simulink model "AcasXuClosedLoop_m_1"  (R2019b)
settings: Solver=VariableStepAuto  StartTime=0.0  StopTime=30  RelTol=1e-3
libraries: neural x1560, simulink x2
(part 2 of 85)

== system AcasXuClosedLoop_m_1/networks/AcasXu_1_1/Layer 5 ==
  "a{4} " : Inport  PortDimensions=50
      mask Display: e = 0.06;c1 = [120 230 180]/255;c2 = ([120 230 180]+0)/(256+128);c3 = ([120 230 180]+128)/(256+128);patch([0 1 1 0],[0 0 1 1],c1);patch([0 1 1 1-e 1-e 0+e],[0 0 1 1-e 0+e 0+e],c2);patch([0 0 1 1-e 0+e 0+e],[0 1 1 1-e 1-e 0+e],c3);plot([0 1 1 0 0],[0 0 1 1 0]);
  Delays 1 : Subsystem
      mask Display: e = 0.06;c1 = [120 150 230]/255;c2 = ([120 150 230]+0)/383;c3 = ([120 150 230]+128)/383;patch([0 1 1 0],[0 0 1 1],c1);patch([0 1 1 1-e 1-e 0+e],[0 0 1 1-e 0+e 0+e],c2);patch([0 0 1 1-e 0+e 0+e],[0 1 1 1-e 1-e 0+e],c3);plot([0 1 1 0 0],[0 0 1 1 0]);disp('0');
  "LW{5,4}" : Subsystem
      mask Display: e = 0.06;c1 = [120 150 230]/255;c2 = ([120 150 230]+0)/383;c3 = ([120 150 230]+128)/383;patch([0 1 1 0],[0 0 1 1],c1);patch([0 1 1 1-e 1-e 0+e],[0 0 1 1-e 0+e 0+e],c2);patch([0 0 1 1-e 0+e 0+e],[0 1 1 1-e 1-e 0+e],c3);plot([0 1 1 0 0],[0 0 1 1 0]);disp('W');
  "b{5}" : Constant  Value=[0.343884000000000022989610215518041513860225677490234375;-0.148704000000000002845723656719201244413852691650390625;-0.182344000000000006078693104427657090127468109130859375;2.092820000000000124629195852321572601795196533203125;0.057392100000000001447375552743324078619480133056640625;1.0727800000000000668620714350254274904727935791015625;-3.537500000000000088817841970012523233890533447265625;0.2902460000000000039932501749717630445957183837890625;1.7852799999999999780442294650129042565822601318359375;0.5703920000000000101181285572238266468048095703125;0.102578000000000002511768570911954157054424285888671875;-0.8676939999999999653113036401919089257717132568359375;-1.8884399999999998964739233997534029185771942138671875;-1.11488999999999993661958797019906342029571533203125;-0.445674999999999987831955650108284316956996917724609375;0.694015999999999966263430906110443174839019775390625;1.2776199999999999779021209178608842194080352783203125;-1.2911200000000000454036808150704018771648406982421875;-1.34224999999999994315658113919198513031005859375;-0.15967100000000000736832816983223892748355865478515625;0.64522299999999999098321268320432864129543304443359375;0.988628999999999980019538270425982773303985595703125;0.5161510000000000264464006249909289181232452392578125;-2.3827400000000000801492205937393009662628173828125;0.67675600000000002420819100734661333262920379638671875;0.76186699999999996091304410583688877522945404052734375;0.056760600000000001330580090552757610566914081573486328125;-0.2224609999999999920827775667930836789309978485107421875;1.869569999999999954098939269897527992725372314453125;1.052049999999999929656269159750081598758697509765625;-0.1076290000000000024460433678541448898613452911376953125;0.0906623000000000012210676914037321694195270538330078125;2.556319999999999925677229839493520557880401611328125;0.87517400000000000748201500755385495722293853759765625;0.08279160000000000685371759345798636786639690399169921875;-1.1624499999999999833022457096376456320285797119140625;1.1968300000000000604671868131845258176326751708984375;0.11945899999999999574473719121670001186430454254150390625;0.052382600000000001383426706524915061891078948974609375;-0.25143999999999999683808482586755417287349700927734375;0.9712009999999999809716655363445170223712921142578125;0.41452299999999997481836544466204941272735595703125;0.55931600000000003536371195878018625080585479736328125;0.71126500000000003609557097661308944225311279296875;-3.244779999999999997584154698415659368038177490234375;0.57999999999999996003197111349436454474925994873046875;0.165872999999999992670751680634566582739353179931640625;-1.2932699999999999196376165855326689779758453369140625;-0.331040999999999974168218841441557742655277252197265625;-0.65416499999999999648281345798750407993793487548828125]
      mask Display: e = 0.06;c1 = [120 150 230]/255;c2 = ([120 150 230]+0)/383;c3 = ([120 150 230]+128)/383;patch([0 1 1 0],[0 0 1 1],c1);patch([0 1 1 1-e 1-e 0+e],[0 0 1 1-e 0+e 0+e],c2);patch([0 0 1 1-e 0+e 0+e],[0 1 1 1-e 1-e 0+e],c3);plot([0 1 1 0 0],[0 0 1 1 0]);disp('b');
  netsum : Sum  Inputs=2  SaturateOnIntegerOverflow=on  InputSameDT=on  OutDataTypeStr=Inherit: Same as first input
      mask Display: e = 0.06;c1 = [120 150 230]/255;c2 = ([120 150 230]+0)/383;c3 = ([120 150 230]+128)/383;patch([0 1 1 0],[0 0 1 1],c1);patch([0 1 1 1-e 1-e 0+e],[0 0 1 1-e 0+e 0+e],c2);patch([0 0 1 1-e 0+e 0+e],[0 1 1 1-e 1-e 0+e],c3);plot([0 1 1 0 0],[0 0 1 1 0]);disp('+');
  tansig : neural/Transfer Functions/tansig
      settings: SourceProductName=Deep Learning Toolbox
  "a{5}" : Outport  InitialOutput=[0;0;0;0;0;0;0;0;0;0;0;0;0;0;0;0;0;0;0;0;0;0;0;0;0;0;0;0;0;0;0;0;0;0;0;0;0;0;0;0;0;0;0;0;0;0;0;0;0;0]
      mask Display: e = 0.06;c1 = [120 230 180]/255;c2 = ([120 230 180]+0)/(256+128);c3 = ([120 230 180]+128)/(256+128);patch([0 1 1 0],[0 0 1 1],c1);patch([0 1 1 1-e 1-e 0+e],[0 0 1 1-e 0+e 0+e],c2);patch([0 0 1 1-e 0+e 0+e],[0 1 1 1-e 1-e 0+e],c3);plot([0 1 1 0 0],[0 0 1 1 0]);
  wires:
  tansig/1 -> "a{5}"/1
  netsum/1 -> tansig/1
  "b{5}"/1 -> netsum/2
  "LW{5,4}"/1("lz{5,4}") -> netsum/1
  Delays 1/1("pd{5,4}") -> "LW{5,4}"/1("ad{5,4}")
  "a{4} "/1 -> Delays 1/1("p{5}")

== system AcasXuClosedLoop_m_1/networks/AcasXu_1_1/Layer 6 ==
  "a{5} " : Inport  PortDimensions=50
      mask Display: e = 0.06;c1 = [120 230 180]/255;c2 = ([120 230 180]+0)/(256+128);c3 = ([120 230 180]+128)/(256+128);patch([0 1 1 0],[0 0 1 1],c1);patch([0 1 1 1-e 1-e 0+e],[0 0 1 1-e 0+e 0+e],c2);patch([0 0 1 1-e 0+e 0+e],[0 1 1 1-e 1-e 0+e],c3);plot([0 1 1 0 0],[0 0 1 1 0]);
  Delays 1 : Subsystem
      mask Display: e = 0.06;c1 = [120 150 230]/255;c2 = ([120 150 230]+0)/383;c3 = ([120 150 230]+128)/383;patch([0 1 1 0],[0 0 1 1],c1);patch([0 1 1 1-e 1-e 0+e],[0 0 1 1-e 0+e 0+e],c2);patch([0 0 1 1-e 0+e 0+e],[0 1 1 1-e 1-e 0+e],c3);plot([0 1 1 0 0],[0 0 1 1 0]);disp('0');
  "LW{6,5}" : Subsystem
      mask Display: e = 0.06;c1 = [120 150 230]/255;c2 = ([120 150 230]+0)/383;c3 = ([120 150 230]+128)/383;patch([0 1 1 0],[0 0 1 1],c1);patch([0 1 1 1-e 1-e 0+e],[0 0 1 1-e 0+e 0+e],c2);patch([0 0 1 1-e 0+e 0+e],[0 1 1 1-e 1-e 0+e],c3);plot([0 1 1 0 0],[0 0 1 1 0]);disp('W');
  "b{6}" : Constant  Value=[-0.4300610000000000265885091721429489552974700927734375;-0.0245742000000000009041212223337424802593886852264404296875;-1.857369999999999965467623042059130966663360595703125;-0.0138151999999999997026378650843980722129344940185546875;0.419246999999999980790477138725691474974155426025390625;-0.2135869999999999990780708003512700088322162628173828125;0.160069999999999990070165267752599902451038360595703125;0.741837999999999997413624441833235323429107666015625;0.0084694499999999998951505375544002163223922252655029296875;-0.72603399999999995717558931573876179754734039306640625;-4.7420600000000003859668140648864209651947021484375;0.069490200000000001967492835319717414677143096923828125;-0.332739999999999980229148377475212328135967254638671875;0.4584289999999999754010104879853315651416778564453125;-1.0340100000000000957101065068854950368404388427734375;-0.436593999999999982097875772524275816977024078369140625;0.08706809999999999549746831917218514718115329742431640625;-1.1747900000000000009237055564881302416324615478515625;0.29503800000000002246025587737676687538623809814453125;0.648179999999999978399500832892954349517822265625;0.59697699999999997988453515063156373798847198486328125;-2.17555999999999993832489053602330386638641357421875;-1.1105899999999999661071115042432211339473724365234375;-0.429719000000000017625012560529285110533237457275390625;0.241839999999999999413802242997917346656322479248046875;0.161131999999999997452704292300040833652019500732421875;0.10325099999999999555999607991907396353781223297119140625;0.1906210000000000126529897670479840599000453948974609375;-2.56280999999999981042719809920527040958404541015625;0.428493999999999986005860819204826839268207550048828125;0.1659190000000000109192654917933396063745021820068359375;-0.041315499999999998059774242165076429955661296844482421875;-3.21201999999999987522869560052640736103057861328125;0.0165723000000000016129764190964124281890690326690673828125;-1.449510000000000076170181273482739925384521484375;-0.212716999999999989423571378210908733308315277099609375;0.096362000000000003208100451956852339208126068115234375;-0.1836109999999999964348518233236973173916339874267578125;-0.55453399999999997138644403094076551496982574462890625;0.33988600000000002143707433788222260773181915283203125;0.366640000000000021440627051561023108661174774169921875;1.1872499999999999165112285481882281601428985595703125;-7.00659999999999971720399116748012602329254150390625;0.8648160000000000291464630208793096244335174560546875;-4.08664999999999967172925607883371412754058837890625;0.1906569999999999931450389567544334568083286285400390625;0.438983999999999985330845220232731662690639495849609375;-0.66478899999999996328625684327562339603900909423828125;-0.1143470000000000041939784978239913471043109893798828125;0.12170599999999999474287193379495874978601932525634765625]
      mask Display: e = 0.06;c1 = [120 150 230]/255;c2 = ([120 150 230]+0)/383;c3 = ([120 150 230]+128)/383;patch([0 1 1 0],[0 0 1 1],c1);patch([0 1 1 1-e 1-e 0+e],[0 0 1 1-e 0+e 0+e],c2);patch([0 0 1 1-e 0+e 0+e],[0 1 1 1-e 1-e 0+e],c3);plot([0 1 1 0 0],[0 0 1 1 0]);disp('b');
  netsum : Sum  Inputs=2  SaturateOnIntegerOverflow=on  InputSameDT=on  OutDataTypeStr=Inherit: Same as first input
      mask Display: e = 0.06;c1 = [120 150 230]/255;c2 = ([120 150 230]+0)/383;c3 = ([120 150 230]+128)/383;patch([0 1 1 0],[0 0 1 1],c1);patch([0 1 1 1-e 1-e 0+e],[0 0 1 1-e 0+e 0+e],c2);patch([0 0 1 1-e 0+e 0+e],[0 1 1 1-e 1-e 0+e],c3);plot([0 1 1 0 0],[0 0 1 1 0]);disp('+');
  tansig : neural/Transfer Functions/tansig
      settings: SourceProductName=Deep Learning Toolbox
  "a{6}" : Outport  InitialOutput=[0;0;0;0;0;0;0;0;0;0;0;0;0;0;0;0;0;0;0;0;0;0;0;0;0;0;0;0;0;0;0;0;0;0;0;0;0;0;0;0;0;0;0;0;0;0;0;0;0;0]
      mask Display: e = 0.06;c1 = [120 230 180]/255;c2 = ([120 230 180]+0)/(256+128);c3 = ([120 230 180]+128)/(256+128);patch([0 1 1 0],[0 0 1 1],c1);patch([0 1 1 1-e 1-e 0+e],[0 0 1 1-e 0+e 0+e],c2);patch([0 0 1 1-e 0+e 0+e],[0 1 1 1-e 1-e 0+e],c3);plot([0 1 1 0 0],[0 0 1 1 0]);
  wires:
  tansig/1 -> "a{6}"/1
  netsum/1 -> tansig/1
  "b{6}"/1 -> netsum/2
  "LW{6,5}"/1("lz{6,5}") -> netsum/1
  Delays 1/1("pd{6,5}") -> "LW{6,5}"/1("ad{6,5}")
  "a{5} "/1 -> Delays 1/1("p{6}")

== system AcasXuClosedLoop_m_1/networks/AcasXu_1_1/Layer 7 ==
  "a{6} " : Inport  PortDimensions=50
      mask Display: e = 0.06;c1 = [120 230 180]/255;c2 = ([120 230 180]+0)/(256+128);c3 = ([120 230 180]+128)/(256+128);patch([0 1 1 0],[0 0 1 1],c1);patch([0 1 1 1-e 1-e 0+e],[0 0 1 1-e 0+e 0+e],c2);patch([0 0 1 1-e 0+e 0+e],[0 1 1 1-e 1-e 0+e],c3);plot([0 1 1 0 0],[0 0 1 1 0]);
  Delays 1 : Subsystem
      mask Display: e = 0.06;c1 = [120 150 230]/255;c2 = ([120 150 230]+0)/383;c3 = ([120 150 230]+128)/383;patch([0 1 1 0],[0 0 1 1],c1);patch([0 1 1 1-e 1-e 0+e],[0 0 1 1-e 0+e 0+e],c2);patch([0 0 1 1-e 0+e 0+e],[0 1 1 1-e 1-e 0+e],c3);plot([0 1 1 0 0],[0 0 1 1 0]);disp('0');
  "LW{7,6}" : Subsystem
      mask Display: e = 0.06;c1 = [120 150 230]/255;c2 = ([120 150 230]+0)/383;c3 = ([120 150 230]+128)/383;patch([0 1 1 0],[0 0 1 1],c1);patch([0 1 1 1-e 1-e 0+e],[0 0 1 1-e 0+e 0+e],c2);patch([0 0 1 1-e 0+e 0+e],[0 1 1 1-e 1-e 0+e],c3);plot([0 1 1 0 0],[0 0 1 1 0]);disp('W');
  "b{7}" : Constant  Value=[-0.01028150000000000070798922280346232582814991474151611328125;-0.01586680000000000034798830483850906603038311004638671875;-0.01548229999999999918769422180275796563364565372467041015625;-0.01533600000000000067312821983023241045884788036346435546875;-0.0148281000000000003080646848729884368367493152618408203125]
      mask Display: e = 0.06;c1 = [120 150 230]/255;c2 = ([120 150 230]+0)/383;c3 = ([120 150 230]+128)/383;patch([0 1 1 0],[0 0 1 1],c1);patch([0 1 1 1-e 1-e 0+e],[0 0 1 1-e 0+e 0+e],c2);patch([0 0 1 1-e 0+e 0+e],[0 1 1 1-e 1-e 0+e],c3);plot([0 1 1 0 0],[0 0 1 1 0]);disp('b');
  netsum : Sum  Inputs=2  SaturateOnIntegerOverflow=on  InputSameDT=on  OutDataTypeStr=Inherit: Same as first input
      mask Display: e = 0.06;c1 = [120 150 230]/255;c2 = ([120 150 230]+0)/383;c3 = ([120 150 230]+128)/383;patch([0 1 1 0],[0 0 1 1],c1);patch([0 1 1 1-e 1-e 0+e],[0 0 1 1-e 0+e 0+e],c2);patch([0 0 1 1-e 0+e 0+e],[0 1 1 1-e 1-e 0+e],c3);plot([0 1 1 0 0],[0 0 1 1 0]);disp('+');
  purelin : neural/Transfer Functions/purelin
      settings: SourceProductName=Deep Learning Toolbox
  "a{7}" : Outport  InitialOutput=[0;0;0;0;0]
      mask Display: e = 0.06;c1 = [120 230 180]/255;c2 = ([120 230 180]+0)/(256+128);c3 = ([120 230 180]+128)/(256+128);patch([0 1 1 0],[0 0 1 1],c1);patch([0 1 1 1-e 1-e 0+e],[0 0 1 1-e 0+e 0+e],c2);patch([0 0 1 1-e 0+e 0+e],[0 1 1 1-e 1-e 0+e],c3);plot([0 1 1 0 0],[0 0 1 1 0]);
  wires:
  purelin/1 -> "a{7}"/1
  netsum/1 -> purelin/1
  "b{7}"/1 -> netsum/2
  "LW{7,6}"/1("lz{7,6}") -> netsum/1
  Delays 1/1("pd{7,6}") -> "LW{7,6}"/1("ad{7,6}")
  "a{6} "/1 -> Delays 1/1("p{7}")

== system AcasXuClosedLoop_m_1/networks/AcasXu_1_1/Process Input 1 ==
  x : Inport  PortDimensions=5
      mask Display: e = 0.06;c1 = [120 230 180]/255;c2 = ([120 230 180]+0)/(256+128);c3 = ([120 230 180]+128)/(256+128);patch([0 1 1 0],[0 0 1 1],c1);patch([0 1 1 1-e 1-e 0+e],[0 0 1 1-e 0+e 0+e],c2);patch([0 0 1 1-e 0+e 0+e],[0 1 1 1-e 1-e 0+e],c3);plot([0 1 1 0 0],[0 0 1 1 0]);
  p : Outport  PortDimensions=5
      mask Display: e = 0.06;c1 = [120 230 180]/255;c2 = ([120 230 180]+0)/(256+128);c3 = ([120 230 180]+128)/(256+128);patch([0 1 1 0],[0 0 1 1],c1);patch([0 1 1 1-e 1-e 0+e],[0 0 1 1-e 0+e 0+e],c2);patch([0 0 1 1-e 0+e 0+e],[0 1 1 1-e 1-e 0+e],c3);plot([0 1 1 0 0],[0 0 1 1 0]);
  wires:
  x/1 -> p/1

== system AcasXuClosedLoop_m_1/networks/AcasXu_1_1/Process Output 1 ==
  a : Inport  PortDimensions=5
      mask Display: e = 0.06;c1 = [120 230 180]/255;c2 = ([120 230 180]+0)/(256+128);c3 = ([120 230 180]+128)/(256+128);patch([0 1 1 0],[0 0 1 1],c1);patch([0 1 1 1-e 1-e 0+e],[0 0 1 1-e 0+e 0+e],c2);patch([0 0 1 1-e 0+e 0+e],[0 1 1 1-e 1-e 0+e],c3);plot([0 1 1 0 0],[0 0 1 1 0]);
  y : Outport  PortDimensions=5
      mask Display: e = 0.06;c1 = [120 230 180]/255;c2 = ([120 230 180]+0)/(256+128);c3 = ([120 230 180]+128)/(256+128);patch([0 1 1 0],[0 0 1 1],c1);patch([0 1 1 1-e 1-e 0+e],[0 0 1 1-e 0+e 0+e],c2);patch([0 0 1 1-e 0+e 0+e],[0 1 1 1-e 1-e 0+e],c3);plot([0 1 1 0 0],[0 0 1 1 0]);
  wires:
  a/1 -> y/1

== system AcasXuClosedLoop_m_1/networks/AcasXu_2_1/Layer 1 ==
  "p{1}" : Inport  PortDimensions=5
      mask Display: e = 0.06;c1 = [120 230 180]/255;c2 = ([120 230 180]+0)/(256+128);c3 = ([120 230 180]+128)/(256+128);patch([0 1 1 0],[0 0 1 1],c1);patch([0 1 1 1-e 1-e 0+e],[0 0 1 1-e 0+e 0+e],c2);patch([0 0 1 1-e 0+e 0+e],[0 1 1 1-e 1-e 0+e],c3);plot([0 1 1 0 0],[0 0 1 1 0]);
  Delays 1 : Subsystem
      mask Display: e = 0.06;c1 = [120 150 230]/255;c2 = ([120 150 230]+0)/383;c3 = ([120 150 230]+128)/383;patch([0 1 1 0],[0 0 1 1],c1);patch([0 1 1 1-e 1-e 0+e],[0 0 1 1-e 0+e 0+e],c2);patch([0 0 1 1-e 0+e 0+e],[0 1 1 1-e 1-e 0+e],c3);plot([0 1 1 0 0],[0 0 1 1 0]);disp('0');
  "IW{1,1}" : Subsystem
      mask Display: e = 0.06;c1 = [120 150 230]/255;c2 = ([120 150 230]+0)/383;c3 = ([120 150 230]+128)/383;patch([0 1 1 0],[0 0 1 1],c1);patch([0 1 1 1-e 1-e 0+e],[0 0 1 1-e 0+e 0+e],c2);patch([0 0 1 1-e 0+e 0+e],[0 1 1 1-e 1-e 0+e],c3);plot([0 1 1 0 0],[0 0 1 1 0]);disp('W');
  "b{1}" : Constant  Value=[0.1625659999999999882902557146735489368438720703125;-0.5818280000000000118376419777632690966129302978515625;-0.8015470000000000094786400950397364795207977294921875;-0.030902499999999999413802242997917346656322479248046875;-0.80615000000000003321787289678468368947505950927734375;-0.044919300000000002281996813735531759448349475860595703125;0.39823100000000000164845914696343243122100830078125;-0.01291710000000000080344619846073328517377376556396484375;-0.15108800000000000007815970093361102044582366943359375;-0.08336590000000000666435795437791966833174228668212890625;0.01728899999999999881339363128063268959522247314453125;0.276963999999999987977616910939104855060577392578125;-0.1317879999999999884874313238469767384231090545654296875;0.1621620000000000005879741138414829038083553314208984375;0.09520820000000000671303013177748653106391429901123046875;-0.50132100000000001660538373471354134380817413330078125;-0.31888600000000000278532752417959272861480712890625;-0.0747223999999999943799622315054875798523426055908203125;-0.467965000000000019841905896100797690451145172119140625;-0.1974539999999999906332703858424792997539043426513671875;-0.12473700000000000065458749531899229623377323150634765625;-0.16273199999999998777155951756867580115795135498046875;-0.0641459000000000056918025848062825389206409454345703125;0.2065120000000000011208811656615580432116985321044921875;-0.2566800000000000192557081390987150371074676513671875;0.1934780000000000110826903210181626491248607635498046875;-0.9121580000000000243431941271410323679447174072265625;0.00345349999999999997257749129175863345153629779815673828125;-0.29590199999999999835864628039416857063770294189453125;-0.7066689999999999916013848633156158030033111572265625;0.051531500000000000916156039920679177157580852508544921875;-0.100573999999999996735056129182339645922183990478515625;-0.11314000000000000445421477479612804017961025238037109375;-0.68570600000000003770850298678851686418056488037109375;-0.75538199999999999789679350215010344982147216796875;0.61229900000000003768008127735811285674571990966796875;0.0901586000000000054033222340876818634569644927978515625;-0.477876000000000022982504788160440512001514434814453125;-0.06931059999999999998721023075631819665431976318359375;-0.63012400000000001742961330819525755941867828369140625;-0.49970700000000001228528390129213221371173858642578125;0.155584000000000000074606987254810519516468048095703125;-0.36052899999999998836841541560715995728969573974609375;0.0822959000000000051588955329862073995172977447509765625;-0.046897899999999999309796550051032681949436664581298828125;0.053298900000000003218669775151283829472959041595458984375;0.44651099999999999123900806807796470820903778076171875;-0.460731999999999974892972431916859932243824005126953125;0.1620850000000000068478556158879655413329601287841796875;-0.6189270000000000049311665861750952899456024169921875]
      mask Display: e = 0.06;c1 = [120 150 230]/255;c2 = ([120 150 230]+0)/383;c3 = ([120 150 230]+128)/383;patch([0 1 1 0],[0 0 1 1],c1);patch([0 1 1 1-e 1-e 0+e],[0 0 1 1-e 0+e 0+e],c2);patch([0 0 1 1-e 0+e 0+e],[0 1 1 1-e 1-e 0+e],c3);plot([0 1 1 0 0],[0 0 1 1 0]);disp('b');
  netsum : Sum  Inputs=2  SaturateOnIntegerOverflow=on  InputSameDT=on  OutDataTypeStr=Inherit: Same as first input
      mask Display: e = 0.06;c1 = [120 150 230]/255;c2 = ([120 150 230]+0)/383;c3 = ([120 150 230]+128)/383;patch([0 1 1 0],[0 0 1 1],c1);patch([0 1 1 1-e 1-e 0+e],[0 0 1 1-e 0+e 0+e],c2);patch([0 0 1 1-e 0+e 0+e],[0 1 1 1-e 1-e 0+e],c3);plot([0 1 1 0 0],[0 0 1 1 0]);disp('+');
  tansig : neural/Transfer Functions/tansig
      settings: SourceProductName=Deep Learning Toolbox
  "a{1}" : Outport  InitialOutput=[0;0;0;0;0;0;0;0;0;0;0;0;0;0;0;0;0;0;0;0;0;0;0;0;0;0;0;0;0;0;0;0;0;0;0;0;0;0;0;0;0;0;0;0;0;0;0;0;0;0]
      mask Display: e = 0.06;c1 = [120 230 180]/255;c2 = ([120 230 180]+0)/(256+128);c3 = ([120 230 180]+128)/(256+128);patch([0 1 1 0],[0 0 1 1],c1);patch([0 1 1 1-e 1-e 0+e],[0 0 1 1-e 0+e 0+e],c2);patch([0 0 1 1-e 0+e 0+e],[0 1 1 1-e 1-e 0+e],c3);plot([0 1 1 0 0],[0 0 1 1 0]);
  wires:
  tansig/1 -> "a{1}"/1
  netsum/1 -> tansig/1
  "b{1}"/1 -> netsum/2
  "IW{1,1}"/1("iz{1,1}") -> netsum/1
  Delays 1/1("pd{1,1}") -> "IW{1,1}"/1("pd{1,1}")
  "p{1}"/1 -> Delays 1/1("p{1}")

== system AcasXuClosedLoop_m_1/networks/AcasXu_2_1/Layer 2 ==
  "a{1} " : Inport  PortDimensions=50
      mask Display: e = 0.06;c1 = [120 230 180]/255;c2 = ([120 230 180]+0)/(256+128);c3 = ([120 230 180]+128)/(256+128);patch([0 1 1 0],[0 0 1 1],c1);patch([0 1 1 1-e 1-e 0+e],[0 0 1 1-e 0+e 0+e],c2);patch([0 0 1 1-e 0+e 0+e],[0 1 1 1-e 1-e 0+e],c3);plot([0 1 1 0 0],[0 0 1 1 0]);
  Delays 1 : Subsystem
      mask Display: e = 0.06;c1 = [120 150 230]/255;c2 = ([120 150 230]+0)/383;c3 = ([120 150 230]+128)/383;patch([0 1 1 0],[0 0 1 1],c1);patch([0 1 1 1-e 1-e 0+e],[0 0 1 1-e 0+e 0+e],c2);patch([0 0 1 1-e 0+e 0+e],[0 1 1 1-e 1-e 0+e],c3);plot([0 1 1 0 0],[0 0 1 1 0]);disp('0');
  "LW{2,1}" : Subsystem
      mask Display: e = 0.06;c1 = [120 150 230]/255;c2 = ([120 150 230]+0)/383;c3 = ([120 150 230]+128)/383;patch([0 1 1 0],[0 0 1 1],c1);patch([0 1 1 1-e 1-e 0+e],[0 0 1 1-e 0+e 0+e],c2);patch([0 0 1 1-e 0+e 0+e],[0 1 1 1-e 1-e 0+e],c3);plot([0 1 1 0 0],[0 0 1 1 0]);disp('W');
  "b{2}" : Constant  Value=[0.552667000000000019355184122105129063129425048828125;-0.6503900000000000236610731008113361895084381103515625;0.7978330000000000143955958264996297657489776611328125;-0.36217500000000002469136006766348145902156829833984375;0.61262600000000000388666876460774801671504974365234375;0.752850000000000019184653865522705018520355224609375;-0.1222810000000000008046896482483134604990482330322265625;-0.004129449999999999787458904165760031901299953460693359375;-0.141452999999999995406341213310952298343181610107421875;-0.656487999999999960465402182308025658130645751953125;0.2476059999999999927666749499621801078319549560546875;-0.0221704999999999992355004252431172062642872333526611328125;0.7398270000000000123918653116561472415924072265625;-0.226283000000000011908696251339279115200042724609375;0.94933999999999996166621940574259497225284576416015625;-0.005919210000000000269915201300818807794712483882904052734375;-0.60101899999999996992983142263256013393402099609375;-0.2269480000000000108340003635021275840699672698974609375;1.03943999999999991956656231195665895938873291015625;-0.056692499999999999837907438404727145098149776458740234375;-0.91461599999999998455990635193302296102046966552734375;0.1633320000000000049578119387660990469157695770263671875;0.304910000000000014352963262354023754596710205078125;-0.70832200000000000716937620381941087543964385986328125;1.278799999999999936761696517351083457469940185546875;1.052869999999999972573050399660132825374603271484375;-0.225430999999999992500221424052142538130283355712890625;-0.2357329999999999980975218250023317523300647735595703125;0.14560899999999998843946968918316997587680816650390625;0.79074999999999995292654375589336268603801727294921875;-0.006529100000000000354749563058476269361563026905059814453125;0.60662000000000004806821607417077757418155670166015625;-0.67515800000000003588951358324266038835048675537109375;0.68973700000000004450839696801267564296722412109375;-0.039575800000000001255262560562186990864574909210205078125;0.026829300000000000370192765331012196838855743408203125;-0.4289330000000000087112539404188282787799835205078125;-0.0243698000000000004894307181757540092803537845611572265625;-1.28910999999999997811528373858891427516937255859375;-0.2416580000000000116866516464142478071153163909912109375;-0.376342000000000009851675031313789077103137969970703125;-0.124746999999999996777688693327945657074451446533203125;-0.287582999999999977536191408944432623684406280517578125;-0.413968999999999975880626834623399190604686737060546875;0.09448620000000000629380991767902742139995098114013671875;0.162760999999999989018562018827651627361774444580078125;-0.340011000000000007670308832530281506478786468505859375;-0.40002999999999999669597627871553413569927215576171875;0.4314810000000000034248159863636828958988189697265625;-1.514089999999999935909045234438963234424591064453125]
      mask Display: e = 0.06;c1 = [120 150 230]/255;c2 = ([120 150 230]+0)/383;c3 = ([120 150 230]+128)/383;patch([0 1 1 0],[0 0 1 1],c1);patch([0 1 1 1-e 1-e 0+e],[0 0 1 1-e 0+e 0+e],c2);patch([0 0 1 1-e 0+e 0+e],[0 1 1 1-e 1-e 0+e],c3);plot([0 1 1 0 0],[0 0 1 1 0]);disp('b');
  netsum : Sum  Inputs=2  SaturateOnIntegerOverflow=on  InputSameDT=on  OutDataTypeStr=Inherit: Same as first input
      mask Display: e = 0.06;c1 = [120 150 230]/255;c2 = ([120 150 230]+0)/383;c3 = ([120 150 230]+128)/383;patch([0 1 1 0],[0 0 1 1],c1);patch([0 1 1 1-e 1-e 0+e],[0 0 1 1-e 0+e 0+e],c2);patch([0 0 1 1-e 0+e 0+e],[0 1 1 1-e 1-e 0+e],c3);plot([0 1 1 0 0],[0 0 1 1 0]);disp('+');
  tansig : neural/Transfer Functions/tansig
      settings: SourceProductName=Deep Learning Toolbox
  "a{2}" : Outport  InitialOutput=[0;0;0;0;0;0;0;0;0;0;0;0;0;0;0;0;0;0;0;0;0;0;0;0;0;0;0;0;0;0;0;0;0;0;0;0;0;0;0;0;0;0;0;0;0;0;0;0;0;0]
      mask Display: e = 0.06;c1 = [120 230 180]/255;c2 = ([120 230 180]+0)/(256+128);c3 = ([120 230 180]+128)/(256+128);patch([0 1 1 0],[0 0 1 1],c1);patch([0 1 1 1-e 1-e 0+e],[0 0 1 1-e 0+e 0+e],c2);patch([0 0 1 1-e 0+e 0+e],[0 1 1 1-e 1-e 0+e],c3);plot([0 1 1 0 0],[0 0 1 1 0]);
  wires:
  tansig/1 -> "a{2}"/1
  netsum/1 -> tansig/1
  "b{2}"/1 -> netsum/2
  "LW{2,1}"/1("lz{2,1}") -> netsum/1
  Delays 1/1("pd{2,1}") -> "LW{2,1}"/1("ad{2,1}")
  "a{1} "/1 -> Delays 1/1("p{2}")

== system AcasXuClosedLoop_m_1/networks/AcasXu_2_1/Layer 3 ==
  "a{2} " : Inport  PortDimensions=50
      mask Display: e = 0.06;c1 = [120 230 180]/255;c2 = ([120 230 180]+0)/(256+128);c3 = ([120 230 180]+128)/(256+128);patch([0 1 1 0],[0 0 1 1],c1);patch([0 1 1 1-e 1-e 0+e],[0 0 1 1-e 0+e 0+e],c2);patch([0 0 1 1-e 0+e 0+e],[0 1 1 1-e 1-e 0+e],c3);plot([0 1 1 0 0],[0 0 1 1 0]);
  Delays 1 : Subsystem
      mask Display: e = 0.06;c1 = [120 150 230]/255;c2 = ([120 150 230]+0)/383;c3 = ([120 150 230]+128)/383;patch([0 1 1 0],[0 0 1 1],c1);patch([0 1 1 1-e 1-e 0+e],[0 0 1 1-e 0+e 0+e],c2);patch([0 0 1 1-e 0+e 0+e],[0 1 1 1-e 1-e 0+e],c3);plot([0 1 1 0 0],[0 0 1 1 0]);disp('0');
  "LW{3,2}" : Subsystem
      mask Display: e = 0.06;c1 = [120 150 230]/255;c2 = ([120 150 230]+0)/383;c3 = ([120 150 230]+128)/383;patch([0 1 1 0],[0 0 1 1],c1);patch([0 1 1 1-e 1-e 0+e],[0 0 1 1-e 0+e 0+e],c2);patch([0 0 1 1-e 0+e 0+e],[0 1 1 1-e 1-e 0+e],c3);plot([0 1 1 0 0],[0 0 1 1 0]);disp('W');
  "b{3}" : Constant  Value=[0.1135380000000000000337507799486047588288784027099609375;-0.4724909999999999943298689686344005167484283447265625;-0.14640500000000000735411731511703692376613616943359375;-0.039939099999999998213962015825018170289695262908935546875;-0.328556999999999987949195201508700847625732421875;-0.284202000000000010171419262405834160745143890380859375;1.0106100000000000083133500083931721746921539306640625;0.611488000000000031519675758318044245243072509765625;0.1767039999999999999591437926937942393124103546142578125;-0.80686599999999997212540847613126970827579498291015625;-0.618649000000000004462208380573429167270660400390625;-0.37239100000000002754774186541908420622348785400390625;-0.7851019999999999665618588551296852529048919677734375;-0.401749999999999996003197111349436454474925994873046875;-0.4810470000000000023732127374387346208095550537109375;-0.399036000000000001808331262509454973042011260986328125;-0.085675200000000006905764848852413706481456756591796875;-1.5937099999999999599964439767063595354557037353515625;-0.87467700000000003779376811507972888648509979248046875;-0.3075390000000000068069994085817597806453704833984375;0.1553900000000000003463895836830488406121730804443359375;-0.2141969999999999985096366117431898601353168487548828125;0.3202059999999999906350467426818795502185821533203125;0.172617999999999993665511510698706842958927154541015625;-1.3244599999999999706545850131078623235225677490234375;0.4562019999999999964046537570538930594921112060546875;-0.30786400000000002652456032592453993856906890869140625;-0.280791999999999986048493383350432850420475006103515625;-0.1406550000000000022470914018413168378174304962158203125;0.342810000000000003606004383982508443295955657958984375;-0.006544570000000000421780388393244720646180212497711181640625;0.10164399999999999824051855057405191473662853240966796875;0.285916000000000003478106691545690409839153289794921875;-0.05973040000000000293578494847679394297301769256591796875;-0.61252399999999995738875213646679185330867767333984375;0.63160300000000002551558964114519767463207244873046875;0.073717599999999994242472212135908193886280059814453125;-0.2241809999999999913899983994269859977066516876220703125;0.357451000000000018719248373599839396774768829345703125;0.8342709999999999848085963094490580260753631591796875;-0.1180340000000000000301980662698042578995227813720703125;-0.0230687000000000010102585434879074455238878726959228515625;1.6209700000000000219557705349870957434177398681640625;0.418847000000000024844126755851902998983860015869140625;-0.5938689999999999802327010911540128290653228759765625;-0.79590799999999994884802845263038761913776397705078125;0.1168619999999999936601824401805060915648937225341796875;0.78231099999999997862687450833618640899658203125;0.86259399999999997188382394597283564507961273193359375;0.61840799999999995772981264963163994252681732177734375]
      mask Display: e = 0.06;c1 = [120 150 230]/255;c2 = ([120 150 230]+0)/383;c3 = ([120 150 230]+128)/383;patch([0 1 1 0],[0 0 1 1],c1);patch([0 1 1 1-e 1-e 0+e],[0 0 1 1-e 0+e 0+e],c2);patch([0 0 1 1-e 0+e 0+e],[0 1 1 1-e 1-e 0+e],c3);plot([0 1 1 0 0],[0 0 1 1 0]);disp('b');
  netsum : Sum  Inputs=2  SaturateOnIntegerOverflow=on  InputSameDT=on  OutDataTypeStr=Inherit: Same as first input
      mask Display: e = 0.06;c1 = [120 150 230]/255;c2 = ([120 150 230]+0)/383;c3 = ([120 150 230]+128)/383;patch([0 1 1 0],[0 0 1 1],c1);patch([0 1 1 1-e 1-e 0+e],[0 0 1 1-e 0+e 0+e],c2);patch([0 0 1 1-e 0+e 0+e],[0 1 1 1-e 1-e 0+e],c3);plot([0 1 1 0 0],[0 0 1 1 0]);disp('+');
  tansig : neural/Transfer Functions/tansig
      settings: SourceProductName=Deep Learning Toolbox
  "a{3}" : Outport  InitialOutput=[0;0;0;0;0;0;0;0;0;0;0;0;0;0;0;0;0;0;0;0;0;0;0;0;0;0;0;0;0;0;0;0;0;0;0;0;0;0;0;0;0;0;0;0;0;0;0;0;0;0]
      mask Display: e = 0.06;c1 = [120 230 180]/255;c2 = ([120 230 180]+0)/(256+128);c3 = ([120 230 180]+128)/(256+128);patch([0 1 1 0],[0 0 1 1],c1);patch([0 1 1 1-e 1-e 0+e],[0 0 1 1-e 0+e 0+e],c2);patch([0 0 1 1-e 0+e 0+e],[0 1 1 1-e 1-e 0+e],c3);plot([0 1 1 0 0],[0 0 1 1 0]);
  wires:
  tansig/1 -> "a{3}"/1
  netsum/1 -> tansig/1
  "b{3}"/1 -> netsum/2
  "LW{3,2}"/1("lz{3,2}") -> netsum/1
  Delays 1/1("pd{3,2}") -> "LW{3,2}"/1("ad{3,2}")
  "a{2} "/1 -> Delays 1/1("p{3}")

== system AcasXuClosedLoop_m_1/networks/AcasXu_2_1/Layer 4 ==
  "a{3} " : Inport  PortDimensions=50
      mask Display: e = 0.06;c1 = [120 230 180]/255;c2 = ([120 230 180]+0)/(256+128);c3 = ([120 230 180]+128)/(256+128);patch([0 1 1 0],[0 0 1 1],c1);patch([0 1 1 1-e 1-e 0+e],[0 0 1 1-e 0+e 0+e],c2);patch([0 0 1 1-e 0+e 0+e],[0 1 1 1-e 1-e 0+e],c3);plot([0 1 1 0 0],[0 0 1 1 0]);
  Delays 1 : Subsystem
      mask Display: e = 0.06;c1 = [120 150 230]/255;c2 = ([120 150 230]+0)/383;c3 = ([120 150 230]+128)/383;patch([0 1 1 0],[0 0 1 1],c1);patch([0 1 1 1-e 1-e 0+e],[0 0 1 1-e 0+e 0+e],c2);patch([0 0 1 1-e 0+e 0+e],[0 1 1 1-e 1-e 0+e],c3);plot([0 1 1 0 0],[0 0 1 1 0]);disp('0');
  "LW{4,3}" : Subsystem
      mask Display: e = 0.06;c1 = [120 150 230]/255;c2 = ([120 150 230]+0)/383;c3 = ([120 150 230]+128)/383;patch([0 1 1 0],[0 0 1 1],c1);patch([0 1 1 1-e 1-e 0+e],[0 0 1 1-e 0+e 0+e],c2);patch([0 0 1 1-e 0+e 0+e],[0 1 1 1-e 1-e 0+e],c3);plot([0 1 1 0 0],[0 0 1 1 0]);disp('W');
  "b{4}" : Constant  Value=[-1.5970800000000000551381162949837744235992431640625;0.1269119999999999970352604350409819744527339935302734375;0.576845000000000052153836804791353642940521240234375;0.2412680000000000102300390381060424260795116424560546875;0.52972699999999994791011204142705537378787994384765625;-1.3435099999999999820232687852694652974605560302734375;-0.022504400000000000792166332530541694723069667816162109375;-1.03296000000000010032863428932614624500274658203125;-1.0873399999999999732125388618442229926586151123046875;-0.39482899999999998552624447256675921380519866943359375;1.1261300000000000753885842641466297209262847900390625;-0.8917880000000000251247911364771425724029541015625;-1.8159199999999999786126636536209844052791595458984375;0.1314599999999999935251793203860870562493801116943359375;0.1503750000000000086597395920762210153043270111083984375;-0.0299447000000000011776801756013810518197715282440185546875;-1.2088699999999998890842789478483609855175018310546875;-1.3006200000000001093525270334794186055660247802734375;0.0253828000000000005009770376318556373007595539093017578125;-1.6926699999999998969002490412094630300998687744140625;-0.382523000000000001907807245515868999063968658447265625;-0.88644000000000000571986902286880649626255035400390625;0.4454919999999999991047161529422737658023834228515625;-1.0608400000000000051869619710487313568592071533203125;-1.2601899999999999213429191513569094240665435791015625;-0.88751800000000002910383045673370361328125;-1.5333900000000000307665004584123380482196807861328125;-0.378825000000000022826185386293218471109867095947265625;0.90598900000000004428812871992704458534717559814453125;-0.49283500000000002305711177541525103151798248291015625;1.0140100000000000779465381128829903900623321533203125;0.98336500000000004462208380573429167270660400390625;0.01440929999999999988613552659444394521415233612060546875;-0.1990520000000000067075234255753457546234130859375;0.48103200000000001512745484433253295719623565673828125;-1.3414900000000000712674363967380486428737640380859375;1.082899999999999973709918776876293122768402099609375;0.6284060000000000201225702767260372638702392578125;-0.47269200000000000105870867628254927694797515869140625;-0.00342631000000000011940226585238633560948073863983154296875;0.621032000000000028450131139834411442279815673828125;-1.3511800000000000476774175695027224719524383544921875;-2.65406999999999992922994351829402148723602294921875;0.147121000000000001772804125721449963748455047607421875;-0.82602900000000001323741116721066646277904510498046875;-0.60095500000000001694644424787838943302631378173828125;0.109816999999999997950084207332110963761806488037109375;0.10649100000000000232347474593552760779857635498046875;0.67279100000000002790301323329913429915904998779296875;-1.3147200000000001107736125049996189773082733154296875]
      mask Display: e = 0.06;c1 = [120 150 230]/255;c2 = ([120 150 230]+0)/383;c3 = ([120 150 230]+128)/383;patch([0 1 1 0],[0 0 1 1],c1);patch([0 1 1 1-e 1-e 0+e],[0 0 1 1-e 0+e 0+e],c2);patch([0 0 1 1-e 0+e 0+e],[0 1 1 1-e 1-e 0+e],c3);plot([0 1 1 0 0],[0 0 1 1 0]);disp('b');
  netsum : Sum  Inputs=2  SaturateOnIntegerOverflow=on  InputSameDT=on  OutDataTypeStr=Inherit: Same as first input
      mask Display: e = 0.06;c1 = [120 150 230]/255;c2 = ([120 150 230]+0)/383;c3 = ([120 150 230]+128)/383;patch([0 1 1 0],[0 0 1 1],c1);patch([0 1 1 1-e 1-e 0+e],[0 0 1 1-e 0+e 0+e],c2);patch([0 0 1 1-e 0+e 0+e],[0 1 1 1-e 1-e 0+e],c3);plot([0 1 1 0 0],[0 0 1 1 0]);disp('+');
  tansig : neural/Transfer Functions/tansig
      settings: SourceProductName=Deep Learning Toolbox
  "a{4}" : Outport  InitialOutput=[0;0;0;0;0;0;0;0;0;0;0;0;0;0;0;0;0;0;0;0;0;0;0;0;0;0;0;0;0;0;0;0;0;0;0;0;0;0;0;0;0;0;0;0;0;0;0;0;0;0]
      mask Display: e = 0.06;c1 = [120 230 180]/255;c2 = ([120 230 180]+0)/(256+128);c3 = ([120 230 180]+128)/(256+128);patch([0 1 1 0],[0 0 1 1],c1);patch([0 1 1 1-e 1-e 0+e],[0 0 1 1-e 0+e 0+e],c2);patch([0 0 1 1-e 0+e 0+e],[0 1 1 1-e 1-e 0+e],c3);plot([0 1 1 0 0],[0 0 1 1 0]);
  wires:
  tansig/1 -> "a{4}"/1
  netsum/1 -> tansig/1
  "b{4}"/1 -> netsum/2
  "LW{4,3}"/1("lz{4,3}") -> netsum/1
  Delays 1/1("pd{4,3}") -> "LW{4,3}"/1("ad{4,3}")
  "a{3} "/1 -> Delays 1/1("p{4}")

== system AcasXuClosedLoop_m_1/networks/AcasXu_2_1/Layer 5 ==
  "a{4} " : Inport  PortDimensions=50
      mask Display: e = 0.06;c1 = [120 230 180]/255;c2 = ([120 230 180]+0)/(256+128);c3 = ([120 230 180]+128)/(256+128);patch([0 1 1 0],[0 0 1 1],c1);patch([0 1 1 1-e 1-e 0+e],[0 0 1 1-e 0+e 0+e],c2);patch([0 0 1 1-e 0+e 0+e],[0 1 1 1-e 1-e 0+e],c3);plot([0 1 1 0 0],[0 0 1 1 0]);
  Delays 1 : Subsystem
      mask Display: e = 0.06;c1 = [120 150 230]/255;c2 = ([120 150 230]+0)/383;c3 = ([120 150 230]+128)/383;patch([0 1 1 0],[0 0 1 1],c1);patch([0 1 1 1-e 1-e 0+e],[0 0 1 1-e 0+e 0+e],c2);patch([0 0 1 1-e 0+e 0+e],[0 1 1 1-e 1-e 0+e],c3);plot([0 1 1 0 0],[0 0 1 1 0]);disp('0');
  "LW{5,4}" : Subsystem
      mask Display: e = 0.06;c1 = [120 150 230]/255;c2 = ([120 150 230]+0)/383;c3 = ([120 150 230]+128)/383;patch([0 1 1 0],[0 0 1 1],c1);patch([0 1 1 1-e 1-e 0+e],[0 0 1 1-e 0+e 0+e],c2);patch([0 0 1 1-e 0+e 0+e],[0 1 1 1-e 1-e 0+e],c3);plot([0 1 1 0 0],[0 0 1 1 0]);disp('W');
  "b{5}" : Constant  Value=[-2.63900999999999985590193318785168230533599853515625;-2.013710000000000110986775325727649033069610595703125;-0.51219400000000003814193405560217797756195068359375;0.64901299999999995105071093348669819533824920654296875;-0.8289560000000000261621835306868888437747955322265625;0.06876459999999999517239501756193931214511394500732421875;-0.77871999999999996777688693327945657074451446533203125;1.6916599999999999415223328469437547028064727783203125;-0.618006999999999973027797750546596944332122802734375;-0.212073000000000011500134178277221508324146270751953125;0.495755000000000001225686219186172820627689361572265625;-1.3396999999999998909316900608246214687824249267578125;-0.0216569999999999991679988653459076886065304279327392578125;0.98979899999999998438937609535059891641139984130859375;0.98598500000000000031974423109204508364200592041015625;0.56454999999999999626965063725947402417659759521484375;-0.61362700000000003353051170051912777125835418701171875;0.1620979999999999920934357078294851817190647125244140625;1.0250600000000000822097945274435915052890777587890625;-0.35661500000000001531219595563015900552272796630859375;-0.33592699999999997562127873607096262276172637939453125;1.0190900000000000513722397954552434384822845458984375;-0.1204709999999999947561946100904606282711029052734375;-0.67662400000000000321875859299325384199619293212890625;0.9827630000000000531912291990010999143123626708984375;1.0297199999999999686650653529795818030834197998046875;1.079120000000000079154460763675160706043243408203125;0.72961799999999998878053020234801806509494781494140625;-1.4112899999999999334221456592786125838756561279296875;1.1897800000000000597566440774244256317615509033203125;1.1006499999999999062083588796667754650115966796875;0.58809100000000003038991280845948494970798492431640625;0.23044100000000000694200252837617881596088409423828125;1.296559999999999934772176857222802937030792236328125;-0.93590399999999995817034914580290205776691436767578125;0.03450509999999999688480301074378076009452342987060546875;-0.0332838000000000022726709403286804445087909698486328125;0.95810099999999998043875848452444188296794891357421875;1.155489999999999906066250332514755427837371826171875;-1.9778800000000000824940116217476315796375274658203125;-0.0857723999999999986432186460660886950790882110595703125;0.9659940000000000193125515579595230519771575927734375;0.79239899999999996449417949406779371201992034912109375;0.447935000000000027586821715885889716446399688720703125;0.7163850000000000495248286824789829552173614501953125;0.83624799999999999133848405108437873423099517822265625;-0.313512999999999986133758511641644872725009918212890625;0.49657899999999999263167183016776107251644134521484375;0.8999580000000000357118778993026353418827056884765625;1.205340000000000078017592386459000408649444580078125]
      mask Display: e = 0.06;c1 = [120 150 230]/255;c2 = ([120 150 230]+0)/383;c3 = ([120 150 230]+128)/383;patch([0 1 1 0],[0 0 1 1],c1);patch([0 1 1 1-e 1-e 0+e],[0 0 1 1-e 0+e 0+e],c2);patch([0 0 1 1-e 0+e 0+e],[0 1 1 1-e 1-e 0+e],c3);plot([0 1 1 0 0],[0 0 1 1 0]);disp('b');
  netsum : Sum  Inputs=2  SaturateOnIntegerOverflow=on  InputSameDT=on  OutDataTypeStr=Inherit: Same as first input
      mask Display: e = 0.06;c1 = [120 150 230]/255;c2 = ([120 150 230]+0)/383;c3 = ([120 150 230]+128)/383;patch([0 1 1 0],[0 0 1 1],c1);patch([0 1 1 1-e 1-e 0+e],[0 0 1 1-e 0+e 0+e],c2);patch([0 0 1 1-e 0+e 0+e],[0 1 1 1-e 1-e 0+e],c3);plot([0 1 1 0 0],[0 0 1 1 0]);disp('+');
  tansig : neural/Transfer Functions/tansig
      settings: SourceProductName=Deep Learning Toolbox
  "a{5}" : Outport  InitialOutput=[0;0;0;0;0;0;0;0;0;0;0;0;0;0;0;0;0;0;0;0;0;0;0;0;0;0;0;0;0;0;0;0;0;0;0;0;0;0;0;0;0;0;0;0;0;0;0;0;0;0]
      mask Display: e = 0.06;c1 = [120 230 180]/255;c2 = ([120 230 180]+0)/(256+128);c3 = ([120 230 180]+128)/(256+128);patch([0 1 1 0],[0 0 1 1],c1);patch([0 1 1 1-e 1-e 0+e],[0 0 1 1-e 0+e 0+e],c2);patch([0 0 1 1-e 0+e 0+e],[0 1 1 1-e 1-e 0+e],c3);plot([0 1 1 0 0],[0 0 1 1 0]);
  wires:
  tansig/1 -> "a{5}"/1
  netsum/1 -> tansig/1
  "b{5}"/1 -> netsum/2
  "LW{5,4}"/1("lz{5,4}") -> netsum/1
  Delays 1/1("pd{5,4}") -> "LW{5,4}"/1("ad{5,4}")
  "a{4} "/1 -> Delays 1/1("p{5}")

== system AcasXuClosedLoop_m_1/networks/AcasXu_2_1/Layer 6 ==
  "a{5} " : Inport  PortDimensions=50
      mask Display: e = 0.06;c1 = [120 230 180]/255;c2 = ([120 230 180]+0)/(256+128);c3 = ([120 230 180]+128)/(256+128);patch([0 1 1 0],[0 0 1 1],c1);patch([0 1 1 1-e 1-e 0+e],[0 0 1 1-e 0+e 0+e],c2);patch([0 0 1 1-e 0+e 0+e],[0 1 1 1-e 1-e 0+e],c3);plot([0 1 1 0 0],[0 0 1 1 0]);
  Delays 1 : Subsystem
      mask Display: e = 0.06;c1 = [120 150 230]/255;c2 = ([120 150 230]+0)/383;c3 = ([120 150 230]+128)/383;patch([0 1 1 0],[0 0 1 1],c1);patch([0 1 1 1-e 1-e 0+e],[0 0 1 1-e 0+e 0+e],c2);patch([0 0 1 1-e 0+e 0+e],[0 1 1 1-e 1-e 0+e],c3);plot([0 1 1 0 0],[0 0 1 1 0]);disp('0');
  "LW{6,5}" : Subsystem
      mask Display: e = 0.06;c1 = [120 150 230]/255;c2 = ([120 150 230]+0)/383;c3 = ([120 150 230]+128)/383;patch([0 1 1 0],[0 0 1 1],c1);patch([0 1 1 1-e 1-e 0+e],[0 0 1 1-e 0+e 0+e],c2);patch([0 0 1 1-e 0+e 0+e],[0 1 1 1-e 1-e 0+e],c3);plot([0 1 1 0 0],[0 0 1 1 0]);disp('W');
  "b{6}" : Constant  Value=[-0.2153650000000000008792966355031239800155162811279296875;-0.062109400000000002106670393686727038584649562835693359375;-0.07159999999999999698019337301957421004772186279296875;-1.48826999999999998181010596454143524169921875;-0.01333860000000000080311313155334573821164667606353759765625;-0.03609310000000000295816704465323709882795810699462890625;-0.838673000000000001818989403545856475830078125;0.0149602999999999992930543868396853213198482990264892578125;-0.239360999999999990439647490347851999104022979736328125;0.059071800000000000696598334570808219723403453826904296875;-0.0638222999999999984765963745303452014923095703125;-0.9191279999999999450466248163138516247272491455078125;-0.40391399999999999526067995248013176023960113525390625;0.1437199999999999866506783519071177579462528228759765625;-2.14405000000000001136868377216160297393798828125;-0.047065500000000003166800155440796515904366970062255859375;0.209419999999999995043964418073301203548908233642578125;-0.03473790000000000210977901815567747689783573150634765625;-0.73888699999999996048671846438082866370677947998046875;-0.02126959999999999961772800816106610000133514404296875;-0.531303999999999998493649400188587605953216552734375;-0.043094399999999997985522526278145960532128810882568359375;-0.1227580000000000060023097603334463201463222503662109375;-0.391701999999999994628296917653642594814300537109375;-0.329054000000000013148593325240653939545154571533203125;-0.0320802000000000031576519177178852260112762451171875;-0.5511470000000000535322897121659480035305023193359375;0.0189694000000000008443468146879240521229803562164306640625;0.041018699999999998218047636555638746358454227447509765625;0.54283000000000003471001264188089407980442047119140625;0.46177400000000001778488467607530765235424041748046875;-0.013170199999999999962430052846684702672064304351806640625;-0.96839200000000003054623221032670699059963226318359375;-0.27990999999999999214850276985089294612407684326171875;-0.7360910000000000508180164615623652935028076171875;-1.158500000000000085265128291212022304534912109375;-1.629599999999999937472239253111183643341064453125;-0.229090999999999989089616292403661645948886871337890625;-0.214002999999999998781419208171428181231021881103515625;-1.2682599999999999429434183184639550745487213134765625;-0.1015729999999999966231456483001238666474819183349609375;-0.3925899999999999945288209346472285687923431396484375;-0.3392399999999999860023081055260263383388519287109375;0.55180200000000001470112920287647284567356109619140625;-0.53329000000000004177991286269389092922210693359375;-0.340164999999999995150545828437316231429576873779296875;0.032162000000000003085975919248085119761526584625244140625;-0.569714999999999971436182022443972527980804443359375;-0.0915195000000000036255443092159111984074115753173828125;0.2293860000000000065600858079051249660551548004150390625]
      mask Display: e = 0.06;c1 = [120 150 230]/255;c2 = ([120 150 230]+0)/383;c3 = ([120 150 230]+128)/383;patch([0 1 1 0],[0 0 1 1],c1);patch([0 1 1 1-e 1-e 0+e],[0 0 1 1-e 0+e 0+e],c2);patch([0 0 1 1-e 0+e 0+e],[0 1 1 1-e 1-e 0+e],c3);plot([0 1 1 0 0],[0 0 1 1 0]);disp('b');
  netsum : Sum  Inputs=2  SaturateOnIntegerOverflow=on  InputSameDT=on  OutDataTypeStr=Inherit: Same as first input
      mask Display: e = 0.06;c1 = [120 150 230]/255;c2 = ([120 150 230]+0)/383;c3 = ([120 150 230]+128)/383;patch([0 1 1 0],[0 0 1 1],c1);patch([0 1 1 1-e 1-e 0+e],[0 0 1 1-e 0+e 0+e],c2);patch([0 0 1 1-e 0+e 0+e],[0 1 1 1-e 1-e 0+e],c3);plot([0 1 1 0 0],[0 0 1 1 0]);disp('+');
  tansig : neural/Transfer Functions/tansig
      settings: SourceProductName=Deep Learning Toolbox
  "a{6}" : Outport  InitialOutput=[0;0;0;0;0;0;0;0;0;0;0;0;0;0;0;0;0;0;0;0;0;0;0;0;0;0;0;0;0;0;0;0;0;0;0;0;0;0;0;0;0;0;0;0;0;0;0;0;0;0]
      mask Display: e = 0.06;c1 = [120 230 180]/255;c2 = ([120 230 180]+0)/(256+128);c3 = ([120 230 180]+128)/(256+128);patch([0 1 1 0],[0 0 1 1],c1);patch([0 1 1 1-e 1-e 0+e],[0 0 1 1-e 0+e 0+e],c2);patch([0 0 1 1-e 0+e 0+e],[0 1 1 1-e 1-e 0+e],c3);plot([0 1 1 0 0],[0 0 1 1 0]);
  wires:
  tansig/1 -> "a{6}"/1
  netsum/1 -> tansig/1
  "b{6}"/1 -> netsum/2
  "LW{6,5}"/1("lz{6,5}") -> netsum/1
  Delays 1/1("pd{6,5}") -> "LW{6,5}"/1("ad{6,5}")
  "a{5} "/1 -> Delays 1/1("p{6}")

== system AcasXuClosedLoop_m_1/networks/AcasXu_2_1/Layer 7 ==
  "a{6} " : Inport  PortDimensions=50
      mask Display: e = 0.06;c1 = [120 230 180]/255;c2 = ([120 230 180]+0)/(256+128);c3 = ([120 230 180]+128)/(256+128);patch([0 1 1 0],[0 0 1 1],c1);patch([0 1 1 1-e 1-e 0+e],[0 0 1 1-e 0+e 0+e],c2);patch([0 0 1 1-e 0+e 0+e],[0 1 1 1-e 1-e 0+e],c3);plot([0 1 1 0 0],[0 0 1 1 0]);
  Delays 1 : Subsystem
      mask Display: e = 0.06;c1 = [120 150 230]/255;c2 = ([120 150 230]+0)/383;c3 = ([120 150 230]+128)/383;patch([0 1 1 0],[0 0 1 1],c1);patch([0 1 1 1-e 1-e 0+e],[0 0 1 1-e 0+e 0+e],c2);patch([0 0 1 1-e 0+e 0+e],[0 1 1 1-e 1-e 0+e],c3);plot([0 1 1 0 0],[0 0 1 1 0]);disp('0');
  "LW{7,6}" : Subsystem
      mask Display: e = 0.06;c1 = [120 150 230]/255;c2 = ([120 150 230]+0)/383;c3 = ([120 150 230]+128)/383;patch([0 1 1 0],[0 0 1 1],c1);patch([0 1 1 1-e 1-e 0+e],[0 0 1 1-e 0+e 0+e],c2);patch([0 0 1 1-e 0+e 0+e],[0 1 1 1-e 1-e 0+e],c3);plot([0 1 1 0 0],[0 0 1 1 0]);disp('W');
  "b{7}" : Constant  Value=[0.08884309999999999429842745257701608352363109588623046875;0.055073799999999999144062456934989313594996929168701171875;0.093211600000000005561417992794304154813289642333984375;0.0427507000000000025874413722704048268496990203857421875;0.0873439000000000020929036281813750974833965301513671875]
      mask Display: e = 0.06;c1 = [120 150 230]/255;c2 = ([120 150 230]+0)/383;c3 = ([120 150 230]+128)/383;patch([0 1 1 0],[0 0 1 1],c1);patch([0 1 1 1-e 1-e 0+e],[0 0 1 1-e 0+e 0+e],c2);patch([0 0 1 1-e 0+e 0+e],[0 1 1 1-e 1-e 0+e],c3);plot([0 1 1 0 0],[0 0 1 1 0]);disp('b');
  netsum : Sum  Inputs=2  SaturateOnIntegerOverflow=on  InputSameDT=on  OutDataTypeStr=Inherit: Same as first input
      mask Display: e = 0.06;c1 = [120 150 230]/255;c2 = ([120 150 230]+0)/383;c3 = ([120 150 230]+128)/383;patch([0 1 1 0],[0 0 1 1],c1);patch([0 1 1 1-e 1-e 0+e],[0 0 1 1-e 0+e 0+e],c2);patch([0 0 1 1-e 0+e 0+e],[0 1 1 1-e 1-e 0+e],c3);plot([0 1 1 0 0],[0 0 1 1 0]);disp('+');
  purelin : neural/Transfer Functions/purelin
      settings: SourceProductName=Deep Learning Toolbox
  "a{7}" : Outport  InitialOutput=[0;0;0;0;0]
      mask Display: e = 0.06;c1 = [120 230 180]/255;c2 = ([120 230 180]+0)/(256+128);c3 = ([120 230 180]+128)/(256+128);patch([0 1 1 0],[0 0 1 1],c1);patch([0 1 1 1-e 1-e 0+e],[0 0 1 1-e 0+e 0+e],c2);patch([0 0 1 1-e 0+e 0+e],[0 1 1 1-e 1-e 0+e],c3);plot([0 1 1 0 0],[0 0 1 1 0]);
  wires:
  purelin/1 -> "a{7}"/1
  netsum/1 -> purelin/1
  "b{7}"/1 -> netsum/2
  "LW{7,6}"/1("lz{7,6}") -> netsum/1
  Delays 1/1("pd{7,6}") -> "LW{7,6}"/1("ad{7,6}")
  "a{6} "/1 -> Delays 1/1("p{7}")

== system AcasXuClosedLoop_m_1/networks/AcasXu_2_1/Process Input 1 ==
  x : Inport  PortDimensions=5
      mask Display: e = 0.06;c1 = [120 230 180]/255;c2 = ([120 230 180]+0)/(256+128);c3 = ([120 230 180]+128)/(256+128);patch([0 1 1 0],[0 0 1 1],c1);patch([0 1 1 1-e 1-e 0+e],[0 0 1 1-e 0+e 0+e],c2);patch([0 0 1 1-e 0+e 0+e],[0 1 1 1-e 1-e 0+e],c3);plot([0 1 1 0 0],[0 0 1 1 0]);
  p : Outport  PortDimensions=5
      mask Display: e = 0.06;c1 = [120 230 180]/255;c2 = ([120 230 180]+0)/(256+128);c3 = ([120 230 180]+128)/(256+128);patch([0 1 1 0],[0 0 1 1],c1);patch([0 1 1 1-e 1-e 0+e],[0 0 1 1-e 0+e 0+e],c2);patch([0 0 1 1-e 0+e 0+e],[0 1 1 1-e 1-e 0+e],c3);plot([0 1 1 0 0],[0 0 1 1 0]);
  wires:
  x/1 -> p/1
